simulink model "MECH6300_PSD_simulink"  (R2020b)
settings: Solver=VariableStepAuto  StartTime=0.0  StopTime=10  RelTol=1e-3
values from neighbouring files (symbols this model uses):
  K = place(A,B,idealPoles)    [MECH6300_PSD.m]    (also in MECH6300_PSE_extra_credit.m = -K)
  K_2 = place(A,B,idealPoles_2)    [MECH6300_PSD.m]    (also in MECH6300_PSE_extra_credit.m = place(A,B,p_f_ideal_2))
libraries: cstblocks x2
settings Model: Creator=Jonas  LastModifiedBy=Jonas

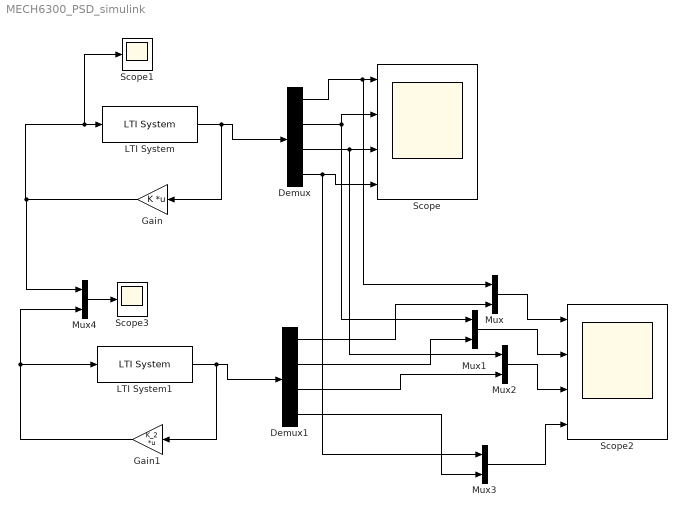
== system MECH6300_PSD_simulink ==
  Demux : Demux
  Demux1 : Demux
  Gain : Gain  Gain=K  Multiplication=Matrix(K*u)
  Gain1 : Gain  Gain=K_2  Multiplication=Matrix(K*u)
  LTI System : cstblocks/LTI System  sys=sys  IC=x0
  LTI System1 : cstblocks/LTI System  sys=sys  IC=x0
  Mux{,1..4} (5 alike) : Mux  Inputs=2
  Scope : Scope  NumInputPorts=4
  Scope1 : Scope
  Scope2 : Scope  NumInputPorts=4
  Scope3 : Scope
  wires:
  LTI System/1 -> Demux/1, Gain/1
  Demux/1 -> Mux/1, Scope/1
  Demux/2 -> Mux1/1, Scope/2
  Demux/3 -> Mux2/1, Scope/3
  Demux/4 -> Mux3/1, Scope/4
  LTI System1/1 -> Demux1/1, Gain1/1
  Demux1/1 -> Mux/2
  Mux/1 -> Scope2/1
  Mux3/1 -> Scope2/4
  Demux1/3 -> Mux2/2
  Mux2/1 -> Scope2/3
  Demux1/2 -> Mux1/2
  Mux1/1 -> Scope2/2
  Demux1/4 -> Mux3/2
  Mux4/1 -> Scope3/1
  Gain/1 -> Mux4/1, Scope1/1, LTI System/1
  Gain1/1 -> Mux4/2, LTI System1/1
